simulink model "MIL4L3_SW6_V1_20220211"  (R2018b)
settings: Solver=FixedStepAuto  StartTime=0.0  StopTime=inf  FixedStep=0.001  RelTol=1e-3
PreLoadFcn:
  | A0_MILtest;
undefined symbols (not defined in the file or in its folder): Clb_ICADirect_LaneDisp_StateFive, Clb_ICADirect_LaneDisp_StateFour, Clb_ICADirect_LaneDisp_StateOne, Clb_ICADirect_LaneDisp_StateThree, Clb_ICADirect_LaneDisp_StateTwo, Clb_ICADirect_LaneDisp_StateZero, Clb_ICADirect_LaneDispSW, Clb_ICADirect_TrnLghtsCom_Switch, Clb_ICADirect_TrnLghtsCom_Value, Clb_ICADirect_TrnLghtsCrtl_Inhb, IMAP_Clb_ACU_Driver_Belt, IMAP_Clb_ACU_Driver_Belt_Over, IMAP_Clb_ACU_Passenger_Belt, IMAP_Clb_ACU_Passenger_Belt_Over, IMAP_Clb_ACU_RearLeft_Belt, IMAP_Clb_ACU_RearLeft_Belt_Over, IMAP_Clb_ACU_RearMiddle_Belt, IMAP_Clb_ACU_RearMiddle_Belt_Over, IMAP_Clb_ACU_RearRight_Belt, IMAP_Clb_ACU_RearRight_Belt_Over, IMAP_Clb_AEB_Switch, IMAP_Clb_AEB_Switch_Over, IMAP_Clb_ALC_TLC_Mode, IMAP_Clb_ALC_TLC_Mode_Over, IMAP_Clb_BCM_Battery_Voltage, IMAP_Clb_BCM_Battery_Voltage_Over, IMAP_Clb_BCM_BrakeLamp_State, IMAP_Clb_BCM_BrakeLamp_State_Over, IMAP_Clb_BCM_CHMSL_Status, IMAP_Clb_BCM_CHMSL_Status_Over, IMAP_Clb_BCM_Door_Lock_State, IMAP_Clb_BCM_Door_Lock_State_Over, IMAP_Clb_BCM_FrontWiper_State, IMAP_Clb_BCM_FrontWiper_State_Over, IMAP_Clb_BCM_FrontWiper_Switch, IMAP_Clb_BCM_FrontWiper_Switch_Over, IMAP_Clb_BCM_HazardLamp, IMAP_Clb_BCM_HazardLamp_Over, IMAP_Clb_BCM_HazardLamp_Switch, IMAP_Clb_BCM_HazardLamp_Switch_Over, IMAP_Clb_BCM_HighBeam_State, IMAP_Clb_BCM_HighBeam_State_Over, IMAP_Clb_BCM_Ignition_State, IMAP_Clb_BCM_Ignition_State_Over, IMAP_Clb_BCM_IHBC_Enabled, IMAP_Clb_BCM_IHBC_Enabled_Over, IMAP_Clb_BCM_Left_Light, IMAP_Clb_BCM_Left_Light_Over, IMAP_Clb_BCM_LeftTurn_Switch, IMAP_Clb_BCM_LeftTurn_Switch_Over, IMAP_Clb_BCM_LF_Door_State, IMAP_Clb_BCM_LF_Door_State_Over, IMAP_Clb_BCM_LowBeam_State, IMAP_Clb_BCM_LowBeam_State_Over, IMAP_Clb_BCM_LR_Door_State, IMAP_Clb_BCM_LR_Door_State_Over, IMAP_Clb_BCM_RF_Door_State, IMAP_Clb_BCM_RF_Door_State_Over, IMAP_Clb_BCM_Right_Light, IMAP_Clb_BCM_Right_Light_Over ... (+547)
libraries: CarMaker4SL x2153, simulink x292, dspstat3 x3, canmsglib x2, simulink_extras x1
(part 9 of 52)

== system MIL4L3_SW6_V1_20220211/CarMaker/VehicleControl/Function/ELK ==
  Bus Selector : BusSelector  OutputSignals=IMAPva_g_ORI_Obj_AbsAx,IMAPva_g_ORI_Obj_AbsAy,IMAPva_g_ORI_Obj_RelVely,IMAPva_g_ORI_Obj_LateralDis,IMAPva_g_ORI_Obj_ExistProb,IMAPva_g_ORI_Obj_ClassProb,IMAPve_d_ORI_L0_ID,IMAPve_g_ORI_L0_ExistProb,IMAPve_g_ORI_L0_TypeConf,IMAPve_d_ORI_R0_ID,IMAPve_g_ORI_R0_ExistProb,IMAPve_g_ORI_R0_TypeConf,IMAPve_d_ORI_L1_ID,IMAPve_g_ORI_L1_ExistProb,IMAPve_g_ORI_L1_TypeConf,IMAPve_d_ORI_R1_ID,IMAPve_g_ORI_R1_ExistProb,IMAPve_g_ORI_R1_TypeConf,IMAPve_d_ORI_RoadedgeL0_ID,IMAPve_g_ORI_RoadedgeL0_ExistProb,IMAPve_g_ORI_RoadedgeL0_C1,IMAPve_g_ORI_RoadedgeL0_C0,IMAPve_g_ORI_RoadedgeL0_C3,IMAPve_g_ORI_RoadedgeL0_C2,IMAPve_d_ORI_RoadedgeL0_Type,IMAPve_d_ORI_RoadedgeR0_ID,IMAPve_g_ORI_RoadedgeR0_ExistProb,IMAPve_g_ORI_RoadedgeR0_C1,IMAPve_g_ORI_RoadedgeR0_C0,IMAPve_g_ORI_RoadedgeR0_C2,IMAPve_g_ORI_RoadedgeR0_C3,IMAPve_d_ORI_RoadedgeR0_Type
  Bus Selector1 : BusSelector  OutputSignals=IMAPve_d_APA_AutoPark_WorkSt,IMAPve_d_ELK_Switch,IMAPve_d_EPS_LKA_State,IMAPve_g_EPS_SW_Trq,IMAPve_g_ESC_LatAcc,IMAPve_g_ESC_YawRate,IMAPve_g_ESC_UnYawRate,IMAPve_g_ESC_VehSpd,IMAPve_g_ESC_LonAcc,IMAPve_g_ESC_Brake_Press,IMAPve_g_SW_Angle,IMAPve_g_SW_Angle_Speed,IMAPve_d_EPS_SteeringAngle_Flag,IMAPve_g_EPS_SteeringAngle,IMAPve_d_EPS_Driver_Override,IMAPve_d_EPS_Driver_Active_ESA,IMAPve_d_BCM_HazardLamp,IMAPve_d_BCM_HazardLamp_Switch,IMAPve_d_BCM_Left_Light,IMAPve_d_BCM_Right_Light,IMAPve_d_BCM_Opening_State,IMAPve_d_BCM_LeftTurn_Switch,IMAPve_d_BCM_RightTurn_Switch,IMAPve_g_EMS_RealPedal,IMAPve_d_TCU_Actual_Gear,IMAPve_d_TCU_Target_Gear,IMAPve_d_BCM_Ignition_State,IMAPve_d_ACU_Driver_Belt,IMAPve_d_SWS_Failure_Status,IMAPve_d_ESC_OFF,IMAPve_d_ESC_AlarmSig,IMAPve_d_ESC_ESC_Active,IMAPve_d_ESC_MSR_Active,IMAPve_d_ESC_TCS_Active,IMAPve_d_ESC_ABS_Active,IMAPve_d_ESC_FL_WheelPulVal,IMAPve_d_ESC_FR_WheelPulVal,IMAPve_d_ESC_RL_WheelPulVal,IMAPve_d_ESC_RR_WheelPulVal,IMAPve_d_ESC_AEB_Active,IMAPve_d_BCM_FrontWiper_State,IMAPve_d_BCM_HighBeam_State,IMAPve_d_ESC_Drive_Direction,IMAPve_d_EPS_Steer_Hold_State,IMAPve_d_Time_System_Clock,IMAPve_d_ORI_CIPV_ID,IMAPve_d_ORI_Obj_Num,IMAPva_d_ORI_Obj_Class,IMAPva_g_ORI_Obj_RelVel,IMAPva_g_ORI_Obj_LongDis,IMAPva_g_ORI_Obj_LAngle,IMAPva_g_ORI_Obj_RAngle,IMAPva_g_ORI_Obj_Width,IMAPva_d_ORI_Obj_ID,IMAPve_g_ORI_L0_C3,IMAPve_g_ORI_L0_C2,IMAPve_g_ORI_L0_C1,IMAPve_g_ORI_L0_C0,IMAPve_d_ORI_L0_Type,IMAPve_g_ORI_L0_VR,IMAPve_g_ORI_L0_W,IMAPve_g_ORI_L1_C3,IMAPve_g_ORI_L1_C2,IMAPve_g_ORI_L1_C1,IMAPve_g_ORI_L1_C0,IMAPve_d_ORI_L1_Type,IMAPve_g_ORI_L1_VR,IMAPve_g_ORI_L1_W,IMAPve_g_ORI_R0_C3,IMAPve_g_ORI_R0_C2,IMAPve_g_ORI_R0_C1,IMAPve_g_ORI_R0_C0,IMAPve_d_ORI_R0_LT,IMAPve_g_ORI_R0_VR,IMAPve_g_ORI_R0_W,IMAPve_g_ORI_R1_C3,IMAPve_g_ORI_R1_C2,IMAPve_g_ORI_R1_C1,IMAPve_g_ORI_R1_C0,IMAPve_d_ORI_R1_LT,IMAPve_g_ORI_R1_VR,IMAPve_g_ORI_R1_W,IMAPve_d_Sensor_Status,IMAPve_d_LF_Radar_Status,IMAPve_d_RF_Radar_Status,IMAPve_d_LR_Radar_Status,IMAPve_d_RR_Radar_Status,IMAPve_d_Fusion_Status,IMAPve_d_Fusion_Time_Stamp,IMAPve_d_obj_Num,IMAPva_d_obj_id,IMAPva_g_obj_pos_x,IMAPva_g_obj_pos_y,IMAPva_g_obj_vel_x,IMAPva_g_obj_vel_y,IMAPva_g_obj_acc_x,IMAPva_g_obj_acc_y,IMAPva_g_obj_pos_var_x,IMAPva_g_obj_pos_var_y,IMAPva_g_obj_pos_var_xy,IMAPva_g_obj_width,IMAPva_g_obj_length,IMAPva_d_obj_class,IMAPva_d_obj_lane,IMAPva_d_obj_status,IMAPva_d_obj_TurnLight,IMAPva_d_obj_BrakeLight,IMAPva_d_obj_MotionStatus,IMAPve_d_Road_Type,IMAPve_g_L0_C0,IMAPve_g_L0_C1,IMAPve_g_L0_C2,IMAPve_g_L0_C3,IMAPve_g_L0_VR,IMAPve_d_L0_Q,IMAPve_d_L0_Type,IMAPve_g_L0_W,IMAPve_g_R0_C0,IMAPve_g_R0_C1,IMAPve_g_R0_C2,IMAPve_g_R0_C3,IMAPve_g_R0_VR,IMAPve_d_R0_Q,IMAPve_d_R0_Type,IMAPve_g_R0_W,IMAPve_g_L1_C0,IMAPve_g_L1_C1,IMAPve_g_L1_C2,IMAPve_g_L1_C3,IMAPve_g_L1_VR,IMAPve_d_L1_Q,IMAPve_d_L1_Type,IMAPve_g_L1_W,IMAPve_g_R1_C0,IMAPve_g_R1_C1,IMAPve_g_R1_C2,IMAPve_g_R1_C3,IMAPve_g_R1_VR,IMAPve_d_R1_Q,IMAPve_d_R1_Type,IMAPve_g_R1_W,IMAPve_g_L0_C0_Back,IMAPve_g_L0_C1_Back,IMAPve_g_L0_C2_Back,IMAPve_g_L0_C3_Back,IMAPve_g_L0_Range_Back,IMAPve_g_R0_C0_Back,IMAPve_g_R0_C1_Back,IMAPve_g_R0_C2_Back,IMAPve_g_R0_C3_Back,IMAPve_g_R0_Range_Back,IMAPve_g_L1_C0_Back,IMAPve_g_L1_C1_Back,IMAPve_g_L1_C2_Back,IMAPve_g_L1_C3_Back,IMAPve_g_L1_Range_Back,IMAPve_g_R1_C0_Back,IMAPve_g_R1_C1_Back,IMAPve_g_R1_C2_Back,IMAPve_g_R1_C3_Back,IMAPve_g_R1_Range_Back,IMAPve_d_Sign_ISA_Value,IMAPve_d_TSR_Sign_Type,IMAPve_g_Camera_Signal_Fault,IMAPve_d_Camera_Status
  Bus Selector2 : BusSelector  OutputSignals=IMAPve_g_Rrg_C0_BACK,IMAPve_g_Rrg_C1_BACK,IMAPve_g_Rrg_C2_BACK,IMAPve_g_Rrg_C3_BACK,IMAPve_g_Rrg_VR_Start_BACK,IMAPve_g_Rrg_VR_End_BACK,IMAPve_d_Rrg_Q_BACK,IMAPve_d_Rrg_TYPE_BACK,IMAPve_g_Lrg_C0_BACK,IMAPve_g_Lrg_C1_BACK,IMAPve_g_Lrg_C2_BACK,IMAPve_g_Lrg_C3_BACK,IMAPve_g_Lrg_VR_Start_BACK,IMAPve_g_Lrg_VR_End_BACK,IMAPve_d_Lrg_Q_BACK,IMAPve_d_Lrg_TYPE_BACK
  Bus Selector6 : BusSelector  OutputSignals=FDMMve_d_ElkFcnConf,FDMMve_d_SignalTStamp
  BusCreator : BusCreator  Inputs=24
  Clock : Clock
  Data Type Conversion : DataTypeConversion
  ELKS : ModelReference  ModelNameDialog=ELKS.slxp  ModelReferenceVersion=1.6  CopyOfModelProtected=on
  tag scope: ELK_output=global
  wires:
  [FDMM_output] -> Bus Selector6/1
  Bus Selector6/1 -> ELKS/1  "<FDMMve_d_ElkFcnConf>"
  Bus Selector6/2 -> ELKS/2  "<FDMMve_d_SignalTStamp>"
  BusCreator/1 -> [ELK_output]
  ELKS/1 -> BusCreator/1  "ELKSve_y_state_ELK_function"
  ELKS/2 -> BusCreator/2  "ELKSve_y_Hands_Off_Warning"
  ELKS/3 -> BusCreator/3  "ELKSve_y_ELK_Action_Indication"
  ELKS/4 -> BusCreator/4  "ELKSve_y_HMI_Popup_Status"
  ELKS/5 -> BusCreator/5  "ELKSve_y_EPS_State_Control"
  ELKS/6 -> BusCreator/6  "ELKSve_g_ELK_SWA_Control"
  ELKS/7 -> BusCreator/7  "ELKSve_g_EPS_Factor_Control"
  ELKS/8 -> BusCreator/8  "ELKSve_y_EPS_ELK_Control"
  ELKS/9 -> BusCreator/9  "ELKSve_y_SignalTStamp"
  ELKS/10 -> BusCreator/10  "ELKSve_y_ELK_VehicleLaneDisp"
  ELKS/11 -> BusCreator/11  "ELKSve_y_ELK_HapticAlarmReq"
  ELKS/12 -> BusCreator/12  "ELKSve_y_ELK_ELKSts"
  ELKS/13 -> BusCreator/13  "ELKSve_y_LKATorqueReq"
  ELKS/14 -> BusCreator/14  "ELKSve_g_LKATorqueReq_Value"
  ELKS/15 -> BusCreator/15  "ELKSve_g_ob9H_10"
  ELKS/16 -> BusCreator/16  "ELKSve_g_ob9L_10"
  ELKS/17 -> BusCreator/17  "ELKSve_g_ob10H_10"
  ELKS/18 -> BusCreator/18  "ELKSve_g_ob10L_10"
  ELKS/19 -> BusCreator/19  "ELKSve_g_ob013H_100"
  ELKS/20 -> BusCreator/20  "ELKSve_g_ob013L_100"
  ELKS/21 -> BusCreator/21  "ELKSve_g_ob014H_100"
  ELKS/22 -> BusCreator/22  "ELKSve_g_ob014L_100"
  ELKS/23 -> BusCreator/23  "ELKSve_g_ob015H_100"
  ELKS/24 -> BusCreator/24  "ELKSve_g_ob015L_100"
  [IMAP_Output] -> Bus Selector1/1, Bus Selector2/1, Bus Selector/1
  Data Type Conversion/1 -> ELKS/168
  Clock/1 -> Data Type Conversion/1  "TIME_System_Clock"
  Bus Selector/8 -> ELKS/176  "<IMAPve_g_ORI_L0_ExistProb>"
  Bus Selector/7 -> ELKS/175  "<IMAPve_d_ORI_L0_ID>"
  Bus Selector/9 -> ELKS/177  "<IMAPve_g_ORI_L0_TypeConf>"
  Bus Selector/6 -> ELKS/174  "<IMAPva_g_ORI_Obj_ClassProb>"
  Bus Selector/10 -> ELKS/178  "<IMAPve_d_ORI_R0_ID>"
  Bus Selector/5 -> ELKS/173  "<IMAPva_g_ORI_Obj_ExistProb>"
  Bus Selector/11 -> ELKS/179  "<IMAPve_g_ORI_R0_ExistProb>"
  Bus Selector/4 -> ELKS/172  "<IMAPva_g_ORI_Obj_LateralDis>"
  Bus Selector/12 -> ELKS/180  "<IMAPve_g_ORI_R0_TypeConf>"
  Bus Selector/3 -> ELKS/171  "<IMAPva_g_ORI_Obj_RelVely>"
  Bus Selector/13 -> ELKS/181  "<IMAPve_d_ORI_L1_ID>"
  Bus Selector/2 -> ELKS/170  "<IMAPva_g_ORI_Obj_AbsAy>"
  Bus Selector/14 -> ELKS/182  "<IMAPve_g_ORI_L1_ExistProb>"
  Bus Selector/1 -> ELKS/169  "<IMAPva_g_ORI_Obj_AbsAx>"
  Bus Selector/15 -> ELKS/183  "<IMAPve_g_ORI_L1_TypeConf>"
  Bus Selector/16 -> ELKS/184  "<IMAPve_d_ORI_R1_ID>"
  Bus Selector/17 -> ELKS/185  "<IMAPve_g_ORI_R1_ExistProb>"
  Bus Selector/18 -> ELKS/186  "<IMAPve_g_ORI_R1_TypeConf>"
  Bus Selector/19 -> ELKS/187  "<IMAPve_d_ORI_RoadedgeL0_ID>"
  Bus Selector/20 -> ELKS/188  "<IMAPve_g_ORI_RoadedgeL0_ExistProb>"
  Bus Selector/21 -> ELKS/189  "<IMAPve_g_ORI_RoadedgeL0_C1>"
  Bus Selector/22 -> ELKS/190  "<IMAPve_g_ORI_RoadedgeL0_C0>"
  Bus Selector/23 -> ELKS/191  "<IMAPve_g_ORI_RoadedgeL0_C3>"
  Bus Selector/24 -> ELKS/192  "<IMAPve_g_ORI_RoadedgeL0_C2>"
  Bus Selector/25 -> ELKS/193  "<IMAPve_d_ORI_RoadedgeL0_Type>"
  Bus Selector/26 -> ELKS/194  "<IMAPve_d_ORI_RoadedgeR0_ID>"
  Bus Selector/27 -> ELKS/195  "<IMAPve_g_ORI_RoadedgeR0_ExistProb>"
  Bus Selector/28 -> ELKS/196  "<IMAPve_g_ORI_RoadedgeR0_C1>"
  Bus Selector/29 -> ELKS/197  "<IMAPve_g_ORI_RoadedgeR0_C0>"
  Bus Selector/32 -> ELKS/200  "<IMAPve_d_ORI_RoadedgeR0_Type>"
  Bus Selector/30 -> ELKS/198  "<IMAPve_g_ORI_RoadedgeR0_C2>"
  Bus Selector/31 -> ELKS/199  "<IMAPve_g_ORI_RoadedgeR0_C3>"
  Bus Selector2/1 -> ELKS/204  "<IMAPve_g_Rrg_C0_BACK>"
  Bus Selector2/2 -> ELKS/205  "<IMAPve_g_Rrg_C1_BACK>"
  Bus Selector2/3 -> ELKS/206  "<IMAPve_g_Rrg_C2_BACK>"
  Bus Selector2/4 -> ELKS/207  "<IMAPve_g_Rrg_C3_BACK>"
  Bus Selector2/5 -> ELKS/208  "<IMAPve_g_Rrg_VR_Start_BACK>"
  Bus Selector2/6 -> ELKS/209  "<IMAPve_g_Rrg_VR_End_BACK>"
  Bus Selector2/7 -> ELKS/210  "<IMAPve_d_Rrg_Q_BACK>"
  Bus Selector2/8 -> ELKS/211  "<IMAPve_d_Rrg_TYPE_BACK>"
  Bus Selector2/9 -> ELKS/212  "<IMAPve_g_Lrg_C0_BACK>"
  Bus Selector2/10 -> ELKS/213  "<IMAPve_g_Lrg_C1_BACK>"
  Bus Selector2/11 -> ELKS/214  "<IMAPve_g_Lrg_C2_BACK>"
  Bus Selector2/12 -> ELKS/215  "<IMAPve_g_Lrg_C3_BACK>"
  Bus Selector2/13 -> ELKS/216  "<IMAPve_g_Lrg_VR_Start_BACK>"
  Bus Selector2/14 -> ELKS/217  "<IMAPve_g_Lrg_VR_End_BACK>"
  Bus Selector2/15 -> ELKS/218  "<IMAPve_d_Lrg_Q_BACK>"
  Bus Selector2/16 -> ELKS/219  "<IMAPve_d_Lrg_TYPE_BACK>"
  ? -> ELKS/203
  ? -> ELKS/202
  ? -> ELKS/201
  Bus Selector1/1 -> ELKS/3  "<IMAPve_d_APA_AutoPark_WorkSt>"
  Bus Selector1/2 -> ELKS/4  "<IMAPve_d_ELK_Switch>"
  Bus Selector1/3 -> ELKS/5  "<IMAPve_d_EPS_LKA_State>"
  Bus Selector1/4 -> ELKS/6  "<IMAPve_g_EPS_SW_Trq>"
  Bus Selector1/5 -> ELKS/7  "<IMAPve_g_ESC_LatAcc>"
  Bus Selector1/6 -> ELKS/8  "<IMAPve_g_ESC_YawRate>"
  Bus Selector1/7 -> ELKS/9  "<IMAPve_g_ESC_UnYawRate>"
  Bus Selector1/8 -> ELKS/10  "<IMAPve_g_ESC_VehSpd>"
  Bus Selector1/9 -> ELKS/11  "<IMAPve_g_ESC_LonAcc>"
  Bus Selector1/10 -> ELKS/12  "<IMAPve_g_ESC_Brake_Press>"
  Bus Selector1/11 -> ELKS/13  "<IMAPve_g_SW_Angle>"
  Bus Selector1/12 -> ELKS/14  "<IMAPve_g_SW_Angle_Speed>"
  Bus Selector1/13 -> ELKS/15  "<IMAPve_d_EPS_SteeringAngle_Flag>"
  Bus Selector1/14 -> ELKS/16  "<IMAPve_g_EPS_SteeringAngle>"
  Bus Selector1/15 -> ELKS/17  "<IMAPve_d_EPS_Driver_Override>"
  Bus Selector1/16 -> ELKS/18  "<IMAPve_d_EPS_Driver_Active_ESA>"
  Bus Selector1/17 -> ELKS/19  "<IMAPve_d_BCM_HazardLamp>"
  Bus Selector1/18 -> ELKS/20  "<IMAPve_d_BCM_HazardLamp_Switch>"
  Bus Selector1/19 -> ELKS/21  "<IMAPve_d_BCM_Left_Light>"
  Bus Selector1/20 -> ELKS/22  "<IMAPve_d_BCM_Right_Light>"
  Bus Selector1/21 -> ELKS/23  "<IMAPve_d_BCM_Opening_State>"
  Bus Selector1/22 -> ELKS/24  "<IMAPve_d_BCM_LeftTurn_Switch>"
  Bus Selector1/23 -> ELKS/25  "<IMAPve_d_BCM_RightTurn_Switch>"
  Bus Selector1/24 -> ELKS/26  "<IMAPve_g_EMS_RealPedal>"
  Bus Selector1/25 -> ELKS/27  "<IMAPve_d_TCU_Actual_Gear>"
  Bus Selector1/26 -> ELKS/28  "<IMAPve_d_TCU_Target_Gear>"
  Bus Selector1/27 -> ELKS/29  "<IMAPve_d_BCM_Ignition_State>"
  Bus Selector1/28 -> ELKS/30  "<IMAPve_d_ACU_Driver_Belt>"
  Bus Selector1/29 -> ELKS/31  "<IMAPve_d_SWS_Failure_Status>"
  Bus Selector1/30 -> ELKS/32  "<IMAPve_d_ESC_OFF>"
  Bus Selector1/31 -> ELKS/33  "<IMAPve_d_ESC_AlarmSig>"
  Bus Selector1/32 -> ELKS/34  "<IMAPve_d_ESC_ESC_Active>"
  Bus Selector1/33 -> ELKS/35  "<IMAPve_d_ESC_MSR_Active>"
  Bus Selector1/34 -> ELKS/36  "<IMAPve_d_ESC_TCS_Active>"
  Bus Selector1/35 -> ELKS/37  "<IMAPve_d_ESC_ABS_Active>"
  Bus Selector1/36 -> ELKS/38  "<IMAPve_d_ESC_FL_WheelPulVal>"
  Bus Selector1/37 -> ELKS/39  "<IMAPve_d_ESC_FR_WheelPulVal>"
  Bus Selector1/38 -> ELKS/40  "<IMAPve_d_ESC_RL_WheelPulVal>"
  Bus Selector1/39 -> ELKS/41  "<IMAPve_d_ESC_RR_WheelPulVal>"
  Bus Selector1/40 -> ELKS/42  "<IMAPve_d_ESC_AEB_Active>"
  Bus Selector1/41 -> ELKS/43  "<IMAPve_d_BCM_FrontWiper_State>"
  Bus Selector1/42 -> ELKS/44  "<IMAPve_d_BCM_HighBeam_State>"
  Bus Selector1/43 -> ELKS/45  "<IMAPve_d_ESC_Drive_Direction>"
  Bus Selector1/44 -> ELKS/46  "<IMAPve_d_EPS_Steer_Hold_State>"
  Bus Selector1/45 -> ELKS/47  "<IMAPve_d_Time_System_Clock>"
  Bus Selector1/46 -> ELKS/48  "<IMAPve_d_ORI_CIPV_ID>"
  Bus Selector1/47 -> ELKS/49  "<IMAPve_d_ORI_Obj_Num>"
  Bus Selector1/48 -> ELKS/50  "<IMAPva_d_ORI_Obj_Class>"
  Bus Selector1/49 -> ELKS/51  "<IMAPva_g_ORI_Obj_RelVel>"
  Bus Selector1/50 -> ELKS/52  "<IMAPva_g_ORI_Obj_LongDis>"
  Bus Selector1/51 -> ELKS/53  "<IMAPva_g_ORI_Obj_LAngle>"
  Bus Selector1/52 -> ELKS/54  "<IMAPva_g_ORI_Obj_RAngle>"
  Bus Selector1/53 -> ELKS/55  "<IMAPva_g_ORI_Obj_Width>"
  Bus Selector1/54 -> ELKS/56  "<IMAPva_d_ORI_Obj_ID>"
  Bus Selector1/55 -> ELKS/57  "<IMAPve_g_ORI_L0_C3>"
  Bus Selector1/56 -> ELKS/58  "<IMAPve_g_ORI_L0_C2>"
  Bus Selector1/57 -> ELKS/59  "<IMAPve_g_ORI_L0_C1>"
  Bus Selector1/58 -> ELKS/60  "<IMAPve_g_ORI_L0_C0>"
  Bus Selector1/59 -> ELKS/61  "<IMAPve_d_ORI_L0_Type>"
  Bus Selector1/60 -> ELKS/62  "<IMAPve_g_ORI_L0_VR>"
  Bus Selector1/61 -> ELKS/63  "<IMAPve_g_ORI_L0_W>"
  Bus Selector1/62 -> ELKS/64  "<IMAPve_g_ORI_L1_C3>"
  Bus Selector1/63 -> ELKS/65  "<IMAPve_g_ORI_L1_C2>"
  Bus Selector1/64 -> ELKS/66  "<IMAPve_g_ORI_L1_C1>"
  Bus Selector1/65 -> ELKS/67  "<IMAPve_g_ORI_L1_C0>"
  Bus Selector1/66 -> ELKS/68  "<IMAPve_d_ORI_L1_Type>"
  Bus Selector1/67 -> ELKS/69  "<IMAPve_g_ORI_L1_VR>"
  Bus Selector1/68 -> ELKS/70  "<IMAPve_g_ORI_L1_W>"
  Bus Selector1/69 -> ELKS/71  "<IMAPve_g_ORI_R0_C3>"
  Bus Selector1/70 -> ELKS/72  "<IMAPve_g_ORI_R0_C2>"
  Bus Selector1/71 -> ELKS/73  "<IMAPve_g_ORI_R0_C1>"
  Bus Selector1/72 -> ELKS/74  "<IMAPve_g_ORI_R0_C0>"
  Bus Selector1/73 -> ELKS/75  "<IMAPve_d_ORI_R0_LT>"
  Bus Selector1/74 -> ELKS/76  "<IMAPve_g_ORI_R0_VR>"
  Bus Selector1/75 -> ELKS/77  "<IMAPve_g_ORI_R0_W>"
  Bus Selector1/76 -> ELKS/78  "<IMAPve_g_ORI_R1_C3>"
  Bus Selector1/77 -> ELKS/79  "<IMAPve_g_ORI_R1_C2>"
  Bus Selector1/78 -> ELKS/80  "<IMAPve_g_ORI_R1_C1>"
  Bus Selector1/79 -> ELKS/81  "<IMAPve_g_ORI_R1_C0>"
  Bus Selector1/80 -> ELKS/82  "<IMAPve_d_ORI_R1_LT>"
  Bus Selector1/81 -> ELKS/83  "<IMAPve_g_ORI_R1_VR>"
  Bus Selector1/82 -> ELKS/84  "<IMAPve_g_ORI_R1_W>"
  Bus Selector1/83 -> ELKS/85  "<IMAPve_d_Sensor_Status>"
  Bus Selector1/84 -> ELKS/86  "<IMAPve_d_LF_Radar_Status>"
  Bus Selector1/85 -> ELKS/87  "<IMAPve_d_RF_Radar_Status>"
  Bus Selector1/86 -> ELKS/88  "<IMAPve_d_LR_Radar_Status>"
  Bus Selector1/87 -> ELKS/89  "<IMAPve_d_RR_Radar_Status>"
  Bus Selector1/88 -> ELKS/90  "<IMAPve_d_Fusion_Status>"
  Bus Selector1/89 -> ELKS/91  "<IMAPve_d_Fusion_Time_Stamp>"
  Bus Selector1/90 -> ELKS/92  "<IMAPve_d_obj_Num>"
  Bus Selector1/91 -> ELKS/93  "<IMAPva_d_obj_id>"
  Bus Selector1/92 -> ELKS/94  "<IMAPva_g_obj_pos_x>"
  Bus Selector1/93 -> ELKS/95  "<IMAPva_g_obj_pos_y>"
  Bus Selector1/94 -> ELKS/96  "<IMAPva_g_obj_vel_x>"
  Bus Selector1/95 -> ELKS/97  "<IMAPva_g_obj_vel_y>"
  Bus Selector1/96 -> ELKS/98  "<IMAPva_g_obj_acc_x>"
  Bus Selector1/97 -> ELKS/99  "<IMAPva_g_obj_acc_y>"
  Bus Selector1/98 -> ELKS/100  "<IMAPva_g_obj_pos_var_x>"
  Bus Selector1/99 -> ELKS/101  "<IMAPva_g_obj_pos_var_y>"
  Bus Selector1/100 -> ELKS/102  "<IMAPva_g_obj_pos_var_xy>"
  Bus Selector1/101 -> ELKS/103  "<IMAPva_g_obj_width>"
  Bus Selector1/102 -> ELKS/104  "<IMAPva_g_obj_length>"
  Bus Selector1/103 -> ELKS/105  "<IMAPva_d_obj_class>"
  Bus Selector1/104 -> ELKS/106  "<IMAPva_d_obj_lane>"
  Bus Selector1/105 -> ELKS/107  "<IMAPva_d_obj_status>"
  Bus Selector1/106 -> ELKS/108  "<IMAPva_d_obj_TurnLight>"
  Bus Selector1/107 -> ELKS/109  "<IMAPva_d_obj_BrakeLight>"
  Bus Selector1/108 -> ELKS/110  "<IMAPva_d_obj_MotionStatus>"
  Bus Selector1/109 -> ELKS/111  "<IMAPve_d_Road_Type>"
  Bus Selector1/110 -> ELKS/112  "<IMAPve_g_L0_C0>"
  Bus Selector1/111 -> ELKS/113  "<IMAPve_g_L0_C1>"
  Bus Selector1/112 -> ELKS/114  "<IMAPve_g_L0_C2>"
  Bus Selector1/113 -> ELKS/115  "<IMAPve_g_L0_C3>"
  Bus Selector1/114 -> ELKS/116  "<IMAPve_g_L0_VR>"
  Bus Selector1/115 -> ELKS/117  "<IMAPve_d_L0_Q>"
  Bus Selector1/116 -> ELKS/118  "<IMAPve_d_L0_Type>"
  Bus Selector1/117 -> ELKS/119  "<IMAPve_g_L0_W>"
  Bus Selector1/118 -> ELKS/120  "<IMAPve_g_R0_C0>"
  Bus Selector1/119 -> ELKS/121  "<IMAPve_g_R0_C1>"
  Bus Selector1/120 -> ELKS/122  "<IMAPve_g_R0_C2>"
  Bus Selector1/121 -> ELKS/123  "<IMAPve_g_R0_C3>"
  Bus Selector1/122 -> ELKS/124  "<IMAPve_g_R0_VR>"
  Bus Selector1/123 -> ELKS/125  "<IMAPve_d_R0_Q>"
  Bus Selector1/124 -> ELKS/126  "<IMAPve_d_R0_Type>"
  Bus Selector1/125 -> ELKS/127  "<IMAPve_g_R0_W>"
  Bus Selector1/126 -> ELKS/128  "<IMAPve_g_L1_C0>"
  Bus Selector1/127 -> ELKS/129  "<IMAPve_g_L1_C1>"
  Bus Selector1/128 -> ELKS/130  "<IMAPve_g_L1_C2>"
  Bus Selector1/129 -> ELKS/131  "<IMAPve_g_L1_C3>"
  Bus Selector1/130 -> ELKS/132  "<IMAPve_g_L1_VR>"
  Bus Selector1/131 -> ELKS/133  "<IMAPve_d_L1_Q>"
  Bus Selector1/132 -> ELKS/134  "<IMAPve_d_L1_Type>"
  Bus Selector1/133 -> ELKS/135  "<IMAPve_g_L1_W>"
  Bus Selector1/134 -> ELKS/136  "<IMAPve_g_R1_C0>"
  Bus Selector1/135 -> ELKS/137  "<IMAPve_g_R1_C1>"
  Bus Selector1/136 -> ELKS/138  "<IMAPve_g_R1_C2>"
  Bus Selector1/137 -> ELKS/139  "<IMAPve_g_R1_C3>"
  Bus Selector1/138 -> ELKS/140  "<IMAPve_g_R1_VR>"
  Bus Selector1/139 -> ELKS/141  "<IMAPve_d_R1_Q>"
  Bus Selector1/140 -> ELKS/142  "<IMAPve_d_R1_Type>"
  Bus Selector1/141 -> ELKS/143  "<IMAPve_g_R1_W>"
  Bus Selector1/142 -> ELKS/144  "<IMAPve_g_L0_C0_Back>"
  Bus Selector1/143 -> ELKS/145  "<IMAPve_g_L0_C1_Back>"
  Bus Selector1/144 -> ELKS/146  "<IMAPve_g_L0_C2_Back>"
  Bus Selector1/145 -> ELKS/147  "<IMAPve_g_L0_C3_Back>"
  Bus Selector1/146 -> ELKS/148  "<IMAPve_g_L0_Range_Back>"
  Bus Selector1/147 -> ELKS/149  "<IMAPve_g_R0_C0_Back>"
  Bus Selector1/148 -> ELKS/150  "<IMAPve_g_R0_C1_Back>"
  Bus Selector1/149 -> ELKS/151  "<IMAPve_g_R0_C2_Back>"
  Bus Selector1/150 -> ELKS/152  "<IMAPve_g_R0_C3_Back>"
  Bus Selector1/151 -> ELKS/153  "<IMAPve_g_R0_Range_Back>"
  Bus Selector1/152 -> ELKS/154  "<IMAPve_g_L1_C0_Back>"
  Bus Selector1/153 -> ELKS/155  "<IMAPve_g_L1_C1_Back>"
  Bus Selector1/154 -> ELKS/156  "<IMAPve_g_L1_C2_Back>"
  Bus Selector1/155 -> ELKS/157  "<IMAPve_g_L1_C3_Back>"
  Bus Selector1/156 -> ELKS/158  "<IMAPve_g_L1_Range_Back>"
  Bus Selector1/157 -> ELKS/159  "<IMAPve_g_R1_C0_Back>"
  Bus Selector1/158 -> ELKS/160  "<IMAPve_g_R1_C1_Back>"
  Bus Selector1/159 -> ELKS/161  "<IMAPve_g_R1_C2_Back>"
  Bus Selector1/160 -> ELKS/162  "<IMAPve_g_R1_C3_Back>"
  Bus Selector1/161 -> ELKS/163  "<IMAPve_g_R1_Range_Back>"
  Bus Selector1/162 -> ELKS/164  "<IMAPve_d_Sign_ISA_Value>"
  Bus Selector1/163 -> ELKS/165  "<IMAPve_d_TSR_Sign_Type>"
  Bus Selector1/164 -> ELKS/166  "<IMAPve_g_Camera_Signal_Fault>"
  Bus Selector1/165 -> ELKS/167  "<IMAPve_d_Camera_Status>"

== system MIL4L3_SW6_V1_20220211/CarMaker/VehicleControl/Function/ESA ==
  Bus Selector : BusSelector  OutputSignals=IMAPve_d_Time_System_Clock,IMAPve_d_ESA_Switch
  Bus Selector1 : BusSelector  OutputSignals=IMAPve_g_EPS_SW_Trq,IMAPve_g_ESC_LonAcc,IMAPve_g_ESC_YawRate,IMAPve_g_ESC_VehSpd,IMAPve_g_ESC_LatAcc,IMAPve_g_ESC_Brake_Press,IMAPve_g_SW_Angle,IMAPve_d_SWS_Failure_Status,IMAPve_g_SW_Angle_Speed,IMAPve_d_TCU_Actual_Gear,IMAPve_d_EPS_LKA_State,IMAPve_d_BCM_HazardLamp,IMAPve_d_BCM_HazardLamp_Switch,IMAPve_d_BCM_Left_Light,IMAPve_d_BCM_Right_Light,IMAPve_d_BCM_Opening_State,IMAPve_d_BCM_Trunk_State,IMAPve_d_BCM_LF_Door_State,IMAPve_d_BCM_RF_Door_State,IMAPve_d_BCM_RR_Door_State,IMAPve_d_BCM_LR_Door_State
  Bus Selector2 : BusSelector  OutputSignals=IMAPve_d_EPS_ESA_State,IMAPve_d_EPS_Driver_Active_ESA,IMAPve_d_EPS_Steer_Hold_State,IMAPve_d_EPS_Driver_Override,IMAPve_d_BCM_Ignition_State,IMAPve_d_ACU_Driver_Belt,IMAPve_d_BCM_FrontWiper_Switch,IMAPve_d_BCM_HighBeam_State,IMAPve_d_APA_AutoPark_WorkSt,IMAPve_d_ESC_AEB_Active,IMAPve_g_EMS_RealPedal,IMAPve_d_ESC_OFF,IMAPve_d_ESC_AlarmSig,IMAPve_d_ESC_ESC_Active,IMAPve_d_ESC_MSR_Active,IMAPve_d_ESC_TCS_Active,IMAPve_d_ESC_ABS_Active,IMAPve_d_ESC_FL_WheelPulVal,IMAPve_d_ESC_FR_WheelPulVal,IMAPve_d_ESC_RL_WheelPulVal,IMAPve_d_ESC_RR_WheelPulVal,IMAPve_d_Sensor_Status,IMAPve_d_LF_Radar_Status,IMAPve_d_RF_Radar_Status,IMAPve_d_LR_Radar_Status,IMAPve_d_RR_Radar_Status,IMAPve_d_Fusion_Status,IMAPve_d_Fusion_Time_Stamp,IMAPve_d_obj_Num,IMAPva_d_obj_id,IMAPva_g_obj_pos_x,IMAPva_g_obj_pos_y,IMAPva_g_obj_vel_x,IMAPva_g_obj_vel_y,IMAPva_g_obj_acc_x,IMAPva_g_obj_acc_y,IMAPva_g_obj_pos_var_x,IMAPva_g_obj_pos_var_y,IMAPva_g_obj_pos_var_xy,IMAPva_g_obj_width,IMAPva_g_obj_length,IMAPva_d_obj_class,IMAPva_d_obj_lane,IMAPva_d_obj_status,IMAPva_d_obj_TurnLight,IMAPva_d_obj_BrakeLight,IMAPva_d_obj_MotionStatus,IMAPve_d_Road_Type,IMAPve_g_L0_C0,IMAPve_g_L0_C1,IMAPve_g_L0_C2,IMAPve_g_L0_C3,IMAPve_g_L0_VR,IMAPve_d_L0_Q,IMAPve_d_L0_Type,IMAPve_g_L0_W,IMAPve_g_R0_C0,IMAPve_g_R0_C1,IMAPve_g_R0_C2,IMAPve_g_R0_C3,IMAPve_g_R0_VR,IMAPve_d_R0_Q,IMAPve_d_R0_Type,IMAPve_g_R0_W,IMAPve_g_L1_C0,IMAPve_g_L1_C1,IMAPve_g_L1_C2,IMAPve_g_L1_C3,IMAPve_g_L1_VR,IMAPve_d_L1_Q,IMAPve_d_L1_Type,IMAPve_g_L1_W,IMAPve_g_R1_C0,IMAPve_g_R1_C1,IMAPve_g_R1_C2,IMAPve_g_R1_C3,IMAPve_g_R1_VR,IMAPve_d_R1_Q,IMAPve_d_R1_Type,IMAPve_g_R1_W,IMAPve_g_L0_C0_Back,IMAPve_g_L0_C1_Back,IMAPve_g_L0_C2_Back,IMAPve_g_L0_C3_Back,IMAPve_g_L0_Range_Back,IMAPve_g_R0_C0_Back,IMAPve_g_R0_C1_Back,IMAPve_g_R0_C2_Back,IMAPve_g_R0_C3_Back,IMAPve_g_R0_Range_Back,IMAPve_g_L1_C0_Back,IMAPve_g_L1_C1_Back,IMAPve_g_L1_C2_Back,IMAPve_g_L1_C3_Back,IMAPve_g_L1_Range_Back,IMAPve_g_R1_C0_Back,IMAPve_g_R1_C1_Back,IMAPve_g_R1_C2_Back,IMAPve_g_R1_C3_Back,IMAPve_g_R1_Range_Back,IMAPve_g_Camera_Signal_Fault
  Bus Selector3 : BusSelector  OutputSignals=IMAPve_d_Camera_State
  Bus Selector4 : BusSelector  OutputSignals=AEBSve_d_AEBAlertReq
  Bus Selector5 : BusSelector  OutputSignals=JABSve_d_AlertReq
  Bus Selector6 : BusSelector  OutputSignals=FDMMve_d_EsaFcnConf,FDMMve_d_SignalTStamp
  Bus Selector7 : BusSelector  OutputSignals=IMAPve_g_Rrg_C0_BACK,IMAPve_g_Rrg_C1_BACK,IMAPve_g_Rrg_C2_BACK,IMAPve_g_Rrg_C3_BACK,IMAPve_g_Rrg_VR_Start_BACK,IMAPve_g_Rrg_VR_End_BACK,IMAPve_d_Rrg_Q_BACK,IMAPve_d_Rrg_TYPE_BACK,IMAPve_g_Lrg_C0_BACK,IMAPve_g_Lrg_C1_BACK,IMAPve_g_Lrg_C2_BACK,IMAPve_g_Lrg_C3_BACK,IMAPve_g_Lrg_VR_Start_BACK,IMAPve_g_Lrg_VR_End_BACK,IMAPve_d_Lrg_Q_BACK,IMAPve_d_Lrg_TYPE_BACK
  BusCreator : BusCreator  Inputs=10
  Clock : Clock
  Data Type Conversion : DataTypeConversion
  Delay : Delay  DelayLength=1
  Delay1 : Delay  DelayLength=1
  ELKS : ModelReference  ModelNameDialog=ESAS.slxp  ModelReferenceVersion=1.6  CopyOfModelProtected=on
  tag scope: ESA_output=global
  wires:
  BusCreator/1 -> [ESA_output]
  ELKS/1 -> BusCreator/1  "ESASve_y_ESA_State"
  ELKS/2 -> BusCreator/2  "ESASve_g_ESA_SWA_CMD"
  ELKS/3 -> BusCreator/3  "ESASve_g_EPS_Factor_Control"
  ELKS/4 -> BusCreator/4  "ESASve_y_SignalTStamp"
  ELKS/5 -> BusCreator/5  "ESASve_y_ESA_FaultSt"
  ELKS/6 -> BusCreator/6  "ESASve_y_ESARequest"
  ELKS/7 -> BusCreator/7  "ESASve_y_ESATorqueReq"
  ELKS/8 -> BusCreator/8  "ESASve_y_LKAActivation"
  [IMAP_Output] -> Bus Selector7/1, Bus Selector3/1, Bus Selector2/1, Bus Selector/1, Bus Selector1/1
  Bus Selector/1 -> ELKS/1  "<IMAPve_d_Time_System_Clock>"
  Bus Selector/2 -> ELKS/2  "<IMAPve_d_ESA_Switch>"
  Bus Selector6/1 -> ELKS/3  "<FDMMve_d_EsaFcnConf>"
  Bus Selector6/2 -> ELKS/4  "<FDMMve_d_SignalTStamp>"
  Data Type Conversion/1 -> ELKS/26
  Bus Selector4/1 -> Delay/1  "<AEBSve_d_AEBAlertReq>"
  Bus Selector5/1 -> Delay1/1  "<JABSve_d_AlertReq>"
  Bus Selector3/1 -> ELKS/130  "<IMAPve_d_Camera_State>"
  [AEB_output] -> Bus Selector4/1
  [JA_output] -> Bus Selector5/1
  [FDMM_output] -> Bus Selector6/1
  Clock/1 -> Data Type Conversion/1  "TIME_System_Clock"
  Bus Selector1/6 -> ELKS/10  "<IMAPve_g_ESC_Brake_Press>"
  Bus Selector1/5 -> ELKS/9  "<IMAPve_g_ESC_LatAcc>"
  Bus Selector1/7 -> ELKS/11  "<IMAPve_g_SW_Angle>"
  Bus Selector1/4 -> ELKS/8  "<IMAPve_g_ESC_VehSpd>"
  Bus Selector1/8 -> ELKS/12  "<IMAPve_d_SWS_Failure_Status>"
  Bus Selector1/3 -> ELKS/7  "<IMAPve_g_ESC_YawRate>"
  Bus Selector1/9 -> ELKS/13  "<IMAPve_g_SW_Angle_Speed>"
  Bus Selector1/2 -> ELKS/6  "<IMAPve_g_ESC_LonAcc>"
  Bus Selector1/10 -> ELKS/14  "<IMAPve_d_TCU_Actual_Gear>"
  Bus Selector1/1 -> ELKS/5  "<IMAPve_g_EPS_SW_Trq>"
  Bus Selector1/11 -> ELKS/15  "<IMAPve_d_EPS_LKA_State>"
  Bus Selector1/12 -> ELKS/16  "<IMAPve_d_BCM_HazardLamp>"
  Bus Selector1/13 -> ELKS/17  "<IMAPve_d_BCM_HazardLamp_Switch>"
  Bus Selector1/14 -> ELKS/18  "<IMAPve_d_BCM_Left_Light>"
  Bus Selector1/15 -> ELKS/19  "<IMAPve_d_BCM_Right_Light>"
  Bus Selector1/16 -> ELKS/20  "<IMAPve_d_BCM_Opening_State>"
  Bus Selector1/17 -> ELKS/21  "<IMAPve_d_BCM_Trunk_State>"
  Bus Selector1/18 -> ELKS/22  "<IMAPve_d_BCM_LF_Door_State>"
  Bus Selector1/19 -> ELKS/23  "<IMAPve_d_BCM_RF_Door_State>"
  Bus Selector1/20 -> ELKS/24  "<IMAPve_d_BCM_RR_Door_State>"
  Bus Selector1/21 -> ELKS/25  "<IMAPve_d_BCM_LR_Door_State>"
  Bus Selector2/1 -> ELKS/27  "<IMAPve_d_EPS_ESA_State>"
  Bus Selector2/2 -> ELKS/28  "<IMAPve_d_EPS_Driver_Active_ESA>"
  Bus Selector2/3 -> ELKS/29  "<IMAPve_d_EPS_Steer_Hold_State>"
  Bus Selector2/4 -> ELKS/30  "<IMAPve_d_EPS_Driver_Override>"
  Bus Selector2/5 -> ELKS/31  "<IMAPve_d_BCM_Ignition_State>"
  Bus Selector2/6 -> ELKS/32  "<IMAPve_d_ACU_Driver_Belt>"
  Bus Selector2/7 -> ELKS/33  "<IMAPve_d_BCM_FrontWiper_Switch>"
  Bus Selector2/8 -> ELKS/34  "<IMAPve_d_BCM_HighBeam_State>"
  Bus Selector2/9 -> ELKS/35  "<IMAPve_d_APA_AutoPark_WorkSt>"
  Bus Selector2/10 -> ELKS/36  "<IMAPve_d_ESC_AEB_Active>"
  Bus Selector2/11 -> ELKS/37  "<IMAPve_g_EMS_RealPedal>"
  Bus Selector2/12 -> ELKS/38  "<IMAPve_d_ESC_OFF>"
  Bus Selector2/13 -> ELKS/39  "<IMAPve_d_ESC_AlarmSig>"
  Bus Selector2/14 -> ELKS/40  "<IMAPve_d_ESC_ESC_Active>"
  Bus Selector2/15 -> ELKS/41  "<IMAPve_d_ESC_MSR_Active>"
  Bus Selector2/16 -> ELKS/42  "<IMAPve_d_ESC_TCS_Active>"
  Bus Selector2/17 -> ELKS/43  "<IMAPve_d_ESC_ABS_Active>"
  Bus Selector2/18 -> ELKS/44  "<IMAPve_d_ESC_FL_WheelPulVal>"
  Bus Selector2/19 -> ELKS/45  "<IMAPve_d_ESC_FR_WheelPulVal>"
  Bus Selector2/20 -> ELKS/46  "<IMAPve_d_ESC_RL_WheelPulVal>"
  Bus Selector2/21 -> ELKS/47  "<IMAPve_d_ESC_RR_WheelPulVal>"
  Bus Selector2/22 -> ELKS/48  "<IMAPve_d_Sensor_Status>"
  Bus Selector2/23 -> ELKS/49  "<IMAPve_d_LF_Radar_Status>"
  Bus Selector2/24 -> ELKS/50  "<IMAPve_d_RF_Radar_Status>"
  Bus Selector2/25 -> ELKS/51  "<IMAPve_d_LR_Radar_Status>"
  Bus Selector2/26 -> ELKS/52  "<IMAPve_d_RR_Radar_Status>"
  Bus Selector2/27 -> ELKS/53  "<IMAPve_d_Fusion_Status>"
  Bus Selector2/28 -> ELKS/54  "<IMAPve_d_Fusion_Time_Stamp>"
  Bus Selector2/29 -> ELKS/55  "<IMAPve_d_obj_Num>"
  Bus Selector2/30 -> ELKS/56  "<IMAPva_d_obj_id>"
  Bus Selector2/31 -> ELKS/57  "<IMAPva_g_obj_pos_x>"
  Bus Selector2/32 -> ELKS/58  "<IMAPva_g_obj_pos_y>"
  Bus Selector2/33 -> ELKS/59  "<IMAPva_g_obj_vel_x>"
  Bus Selector2/34 -> ELKS/60  "<IMAPva_g_obj_vel_y>"
  Bus Selector2/35 -> ELKS/61  "<IMAPva_g_obj_acc_x>"
  Bus Selector2/36 -> ELKS/62  "<IMAPva_g_obj_acc_y>"
  Bus Selector2/37 -> ELKS/63  "<IMAPva_g_obj_pos_var_x>"
  Bus Selector2/38 -> ELKS/64  "<IMAPva_g_obj_pos_var_y>"
  Bus Selector2/39 -> ELKS/65  "<IMAPva_g_obj_pos_var_xy>"
  Bus Selector2/40 -> ELKS/66  "<IMAPva_g_obj_width>"
  Bus Selector2/41 -> ELKS/67  "<IMAPva_g_obj_length>"
  Bus Selector2/42 -> ELKS/68  "<IMAPva_d_obj_class>"
  Bus Selector2/43 -> ELKS/69  "<IMAPva_d_obj_lane>"
  Bus Selector2/44 -> ELKS/70  "<IMAPva_d_obj_status>"
  Bus Selector2/45 -> ELKS/71  "<IMAPva_d_obj_TurnLight>"
  Bus Selector2/46 -> ELKS/72  "<IMAPva_d_obj_BrakeLight>"
  Bus Selector2/47 -> ELKS/73  "<IMAPva_d_obj_MotionStatus>"
  Bus Selector2/48 -> ELKS/74  "<IMAPve_d_Road_Type>"
  Bus Selector2/49 -> ELKS/75  "<IMAPve_g_L0_C0>"
  Bus Selector2/50 -> ELKS/76  "<IMAPve_g_L0_C1>"
  Bus Selector2/51 -> ELKS/77  "<IMAPve_g_L0_C2>"
  Bus Selector2/52 -> ELKS/78  "<IMAPve_g_L0_C3>"
  Bus Selector2/53 -> ELKS/79  "<IMAPve_g_L0_VR>"
  Bus Selector2/54 -> ELKS/80  "<IMAPve_d_L0_Q>"
  Bus Selector2/55 -> ELKS/81  "<IMAPve_d_L0_Type>"
  Bus Selector2/56 -> ELKS/82  "<IMAPve_g_L0_W>"
  Bus Selector2/57 -> ELKS/83  "<IMAPve_g_R0_C0>"
  Bus Selector2/58 -> ELKS/84  "<IMAPve_g_R0_C1>"
  Bus Selector2/59 -> ELKS/85  "<IMAPve_g_R0_C2>"
  Bus Selector2/60 -> ELKS/86  "<IMAPve_g_R0_C3>"
  Bus Selector2/61 -> ELKS/87  "<IMAPve_g_R0_VR>"
  Bus Selector2/62 -> ELKS/88  "<IMAPve_d_R0_Q>"
  Bus Selector2/63 -> ELKS/89  "<IMAPve_d_R0_Type>"
  Bus Selector2/64 -> ELKS/90  "<IMAPve_g_R0_W>"
  Bus Selector2/65 -> ELKS/91  "<IMAPve_g_L1_C0>"
  Bus Selector2/66 -> ELKS/92  "<IMAPve_g_L1_C1>"
  Bus Selector2/67 -> ELKS/93  "<IMAPve_g_L1_C2>"
  Bus Selector2/68 -> ELKS/94  "<IMAPve_g_L1_C3>"
  Bus Selector2/69 -> ELKS/95  "<IMAPve_g_L1_VR>"
  Bus Selector2/70 -> ELKS/96  "<IMAPve_d_L1_Q>"
  Bus Selector2/71 -> ELKS/97  "<IMAPve_d_L1_Type>"
  Bus Selector2/72 -> ELKS/98  "<IMAPve_g_L1_W>"
  Bus Selector2/73 -> ELKS/99  "<IMAPve_g_R1_C0>"
  Bus Selector2/74 -> ELKS/100  "<IMAPve_g_R1_C1>"
  Bus Selector2/75 -> ELKS/101  "<IMAPve_g_R1_C2>"
  Bus Selector2/76 -> ELKS/102  "<IMAPve_g_R1_C3>"
  Bus Selector2/77 -> ELKS/103  "<IMAPve_g_R1_VR>"
  Bus Selector2/78 -> ELKS/104  "<IMAPve_d_R1_Q>"
  Bus Selector2/79 -> ELKS/105  "<IMAPve_d_R1_Type>"
  Bus Selector2/80 -> ELKS/106  "<IMAPve_g_R1_W>"
  Bus Selector2/81 -> ELKS/107  "<IMAPve_g_L0_C0_Back>"
  Bus Selector2/82 -> ELKS/108  "<IMAPve_g_L0_C1_Back>"
  Bus Selector2/83 -> ELKS/109  "<IMAPve_g_L0_C2_Back>"
  Bus Selector2/84 -> ELKS/110  "<IMAPve_g_L0_C3_Back>"
  Bus Selector2/85 -> ELKS/111  "<IMAPve_g_L0_Range_Back>"
  Bus Selector2/86 -> ELKS/112  "<IMAPve_g_R0_C0_Back>"
  Bus Selector2/87 -> ELKS/113  "<IMAPve_g_R0_C1_Back>"
  Bus Selector2/88 -> ELKS/114  "<IMAPve_g_R0_C2_Back>"
  Bus Selector2/89 -> ELKS/115  "<IMAPve_g_R0_C3_Back>"
  Bus Selector2/90 -> ELKS/116  "<IMAPve_g_R0_Range_Back>"
  Bus Selector2/91 -> ELKS/117  "<IMAPve_g_L1_C0_Back>"
  Bus Selector2/92 -> ELKS/118  "<IMAPve_g_L1_C1_Back>"
  Bus Selector2/93 -> ELKS/119  "<IMAPve_g_L1_C2_Back>"
  Bus Selector2/94 -> ELKS/120  "<IMAPve_g_L1_C3_Back>"
  Bus Selector2/95 -> ELKS/121  "<IMAPve_g_L1_Range_Back>"
  Bus Selector2/96 -> ELKS/122  "<IMAPve_g_R1_C0_Back>"
  Bus Selector2/97 -> ELKS/123  "<IMAPve_g_R1_C1_Back>"
  Bus Selector2/98 -> ELKS/124  "<IMAPve_g_R1_C2_Back>"
  Bus Selector2/99 -> ELKS/125  "<IMAPve_g_R1_C3_Back>"
  Bus Selector2/100 -> ELKS/126  "<IMAPve_g_R1_Range_Back>"
  Bus Selector2/101 -> ELKS/127  "<IMAPve_g_Camera_Signal_Fault>"
  Bus Selector7/1 -> ELKS/134  "<IMAPve_g_Rrg_C0_BACK>"
  Bus Selector7/2 -> ELKS/135  "<IMAPve_g_Rrg_C1_BACK>"
  Bus Selector7/3 -> ELKS/136  "<IMAPve_g_Rrg_C2_BACK>"
  Bus Selector7/4 -> ELKS/137  "<IMAPve_g_Rrg_C3_BACK>"
  Bus Selector7/5 -> ELKS/138  "<IMAPve_g_Rrg_VR_Start_BACK>"
  Bus Selector7/6 -> ELKS/139  "<IMAPve_g_Rrg_VR_End_BACK>"
  Bus Selector7/7 -> ELKS/140  "<IMAPve_d_Rrg_Q_BACK>"
  Bus Selector7/8 -> ELKS/141  "<IMAPve_d_Rrg_TYPE_BACK>"
  Bus Selector7/9 -> ELKS/142  "<IMAPve_g_Lrg_C0_BACK>"
  Bus Selector7/10 -> ELKS/143  "<IMAPve_g_Lrg_C1_BACK>"
  Bus Selector7/11 -> ELKS/144  "<IMAPve_g_Lrg_C2_BACK>"
  Bus Selector7/12 -> ELKS/145  "<IMAPve_g_Lrg_C3_BACK>"
  Bus Selector7/13 -> ELKS/146  "<IMAPve_g_Lrg_VR_Start_BACK>"
  Bus Selector7/14 -> ELKS/147  "<IMAPve_g_Lrg_VR_End_BACK>"
  Bus Selector7/15 -> ELKS/148  "<IMAPve_d_Lrg_Q_BACK>"
  Bus Selector7/16 -> ELKS/149  "<IMAPve_d_Lrg_TYPE_BACK>"
  ELKS/9 -> BusCreator/9  "ICABve_g_ob012H_100"
  ELKS/10 -> BusCreator/10  "ICABve_g_ob012L_100"
  Delay/1 -> ELKS/128  "AEBS_AEBAlertReq"
  Delay1/1 -> ELKS/129  "JABS_AlertReq"

== system MIL4L3_SW6_V1_20220211/CarMaker/VehicleControl/Function/FDMM ==
  note: 输入新增8，输出删除1
  Bus Selector : BusSelector  OutputSignals=IMAPve_d_LKA_Main_Switch,IMAPve_d_LKA_Mode,IMAPve_d_AEB_Switch,IMAPve_d_FCW_Switch,IMAPve_d_FCW_Sensitivity,IMAPve_d_ISA_Switch,IMAPve_d_TSR_Switch,IMAPve_d_ISA_ISLC_Mode,IMAPve_d_LDW_Warn_Mode,IMAPve_d_SCC_Left_SwitchSig,IMAPve_d_ALC_TLC_Mode,IMAPve_d_Speed_Limit,IMAPve_d_ESA_Switch,IMAPve_d_ELK_Switch,IMAPve_d_PEPS_RKE_Command,IMAPve_d_BSD_LCW_Switch,IMAPve_d_FCTA_Switch,IMAPve_d_RCTA_Swtich,IMAPve_d_DOW_Switch,IMAPve_d_JA_Brake_Switch,IMAPve_d_JA_Alert_Switch,IMAPve_d_APA_AutoPark_WorkSt,IMAPve_d_Radar_State,IMAPve_d_Camera_State,IMAPve_d_Sensor_Status,IMAPve_d_LF_Radar_Status,IMAPve_d_RF_Radar_Status,IMAPve_d_LR_Radar_Status,IMAPve_d_RR_Radar_Status,IMAPve_d_Fusion_Status
  Bus Selector1 : BusSelector  OutputSignals=JABSve_d_DbFunFARCSta
  Bus Selector2 : BusSelector  Commented=on  OutputSignals=ELKSve_y_state_ELK_function
  Bus Selector3 : BusSelector  Commented=on  OutputSignals=ESASve_y_ESA_State
  Bus Selector4 : BusSelector  Commented=on  OutputSignals=AEBSve_d_AEBAlertReq
  Bus Selector5 : BusSelector  Commented=on  OutputSignals=ICABve_d_ICAMode,ICABve_d_ICAState
  Bus Selector6 : BusSelector  OutputSignals=LKASve_y_EPS_State_Control
  Bus Selector7 : BusSelector  Commented=on  OutputSignals=ACCSve_d_ACC_State
  Bus Selector11 : BusSelector  OutputSignals=FDMMve_d_AccFcnConf
  BusCreator : BusCreator  Inputs=10
  Clock1 : Clock
  Data Type  Conversion511 : DataTypeConversion
  Data Type Conversion : DataTypeConversion
  From2 : From  Commented=on  GotoTag=ELK_output
  From3 : From  Commented=on  GotoTag=ESA_output
  From4 : From  Commented=on  GotoTag=AEB_output
  From5 : From  Commented=on  GotoTag=ICAB_output
  From7 : From  Commented=on  GotoTag=ACC_output
  Model1 : ModelReference  ModelNameDialog=FDMM.slxp  ModelReferenceVersion=1.5  CopyOfModelProtected=on
  Rate Transition : RateTransition  OutPortSampleTime=0.001
  tag scope: FDMM_output=global, FDMMve_d_AccFcnConf=global
  wires:
  Model1/10 -> BusCreator/10  "FDMMve_d_SignalTStamp"
  Rate Transition/1 -> Data Type  Conversion511/1
  Clock1/1 -> Rate Transition/1
  Model1/1 -> BusCreator/1  "FDMMve_d_JaFcnConf"
  Model1/2 -> BusCreator/2  "FDMMve_d_AebFcnConf"
  Model1/3 -> BusCreator/3  "FDMMve_d_EsaFcnConf"
  Model1/4 -> BusCreator/4  "FDMMve_d_ElkFcnConf"
  Model1/8 -> BusCreator/8  "FDMMve_d_EwFcnConf"
  Model1/5 -> BusCreator/5  "FDMMve_d_LkaFcnConf"
  Model1/6 -> BusCreator/6  "FDMMve_d_IcaFcnConf"
  Model1/7 -> BusCreator/7  "FDMMve_d_AccFcnConf"
  Data Type Conversion/1 -> BusCreator/9  "FDMMve_g_Adas2Fapa"
  Bus Selector11/1 -> [FDMMve_d_AccFcnConf]  "<FDMMve_d_AccFcnConf>"
  BusCreator/1 -> Bus Selector11/1, [FDMM_output]
  [IMAP_Output] -> Bus Selector/1
  Model1/9 -> Data Type Conversion/1
  Bus Selector/10 -> Model1/11  "<IMAPve_d_SCC_Left_SwitchSig>"
  Bus Selector/9 -> Model1/10  "<IMAPve_d_LDW_Warn_Mode>"
  Bus Selector/11 -> Model1/12  "<IMAPve_d_ALC_TLC_Mode>"
  Bus Selector/8 -> Model1/9  "<IMAPve_d_ISA_ISLC_Mode>"
  Bus Selector/12 -> Model1/13  "<IMAPve_d_Speed_Limit>"
  Bus Selector/7 -> Model1/8  "<IMAPve_d_TSR_Switch>"
  Bus Selector/13 -> Model1/14  "<IMAPve_d_ESA_Switch>"
  Bus Selector/6 -> Model1/7  "<IMAPve_d_ISA_Switch>"
  Bus Selector/5 -> Model1/6  "<IMAPve_d_FCW_Sensitivity>"
  Bus Selector/4 -> Model1/5  "<IMAPve_d_FCW_Switch>"
  Bus Selector/3 -> Model1/4  "<IMAPve_d_AEB_Switch>"
  Bus Selector/2 -> Model1/3  "<IMAPve_d_LKA_Mode>"
  Bus Selector/1 -> Model1/2  "<IMAPve_d_LKA_Main_Switch>"
  Data Type  Conversion511/1 -> Model1/1
  Bus Selector/14 -> Model1/15  "<IMAPve_d_ELK_Switch>"
  Bus Selector/15 -> Model1/16  "<IMAPve_d_PEPS_RKE_Command>"
  Bus Selector/16 -> Model1/17  "<IMAPve_d_BSD_LCW_Switch>"
  Bus Selector/17 -> Model1/18  "<IMAPve_d_FCTA_Switch>"
  Bus Selector/18 -> Model1/19  "<IMAPve_d_RCTA_Swtich>"
  Bus Selector/19 -> Model1/20  "<IMAPve_d_DOW_Switch>"
  Bus Selector/20 -> Model1/21  "<IMAPve_d_JA_Brake_Switch>"
  Bus Selector/21 -> Model1/22  "<IMAPve_d_JA_Alert_Switch>"
  Bus Selector/22 -> Model1/23  "<IMAPve_d_APA_AutoPark_WorkSt>"
  Bus Selector/23 -> Model1/24  "<IMAPve_d_Radar_State>"
  Bus Selector/24 -> Model1/25  "<IMAPve_d_Camera_State>"
  Bus Selector/25 -> Model1/26  "<IMAPve_d_Sensor_Status>"
  Bus Selector/26 -> Model1/27  "<IMAPve_d_LF_Radar_Status>"
  Bus Selector/27 -> Model1/28  "<IMAPve_d_RF_Radar_Status>"
  Bus Selector/28 -> Model1/29  "<IMAPve_d_LR_Radar_Status>"
  Bus Selector/29 -> Model1/30  "<IMAPve_d_RR_Radar_Status>"
  Bus Selector/30 -> Model1/31  "<IMAPve_d_Fusion_Status>"
  [JA_output] -> Bus Selector1/1
  Bus Selector1/1 -> Model1/32  "<JABSve_d_DbFunFARCSta>"
  From2/1 -> Bus Selector2/1
  Bus Selector2/1 -> Model1/33  "<ELKSve_y_state_ELK_function>"
  From3/1 -> Bus Selector3/1
  Bus Selector3/1 -> Model1/34  "<ESASve_y_ESA_State>"
  From4/1 -> Bus Selector4/1
  Bus Selector4/1 -> Model1/35  "<AEBSve_d_AEBAlertReq>"
  From5/1 -> Bus Selector5/1
  Bus Selector5/1 -> Model1/36  "<ICABve_d_ICAMode>"
  Bus Selector5/2 -> Model1/37  "<ICABve_d_ICAState>"
  [LKA_output] -> Bus Selector6/1
  Bus Selector6/1 -> Model1/38  "<LKASve_y_EPS_State_Control>"
  From7/1 -> Bus Selector7/1
  Bus Selector7/1 -> Model1/39  "<ACCSve_d_ACC_State>"
